simulink subsystem "PumpEfficiency"  (R2019b)
settings: Solver=VariableStepAuto  StartTime=0.0  StopTime=10.0  RelTol=1e-3
values from neighbouring files (symbols this model uses):
  keta = 8e-5    (= 8e-05)    [part1.m]
settings Model: Creator=ovi  LastModifiedBy=ovi

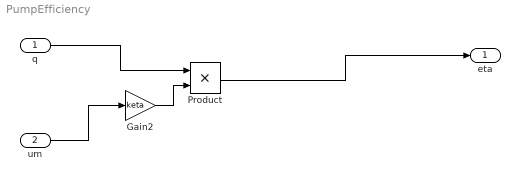
== system PumpEfficiency ==
  q : Inport
  "um " : Inport  Port=2
  Gain2 : Gain  Gain=keta
  Product : Product
  eta : Outport
  wires:
  q/1 -> Product/1
  "um "/1 -> Gain2/1
  Gain2/1 -> Product/2
  Product/1 -> eta/1
